simulink subsystem "Colision"  (R2024b)
settings: Solver=VariableStepAuto  StartTime=0.0  StopTime=10.0  RelTol=1e-3
libraries: simulink x4, arduinosensorlib x3
settings Model: Creator=Chenfu  LastModifiedBy=Chenfu

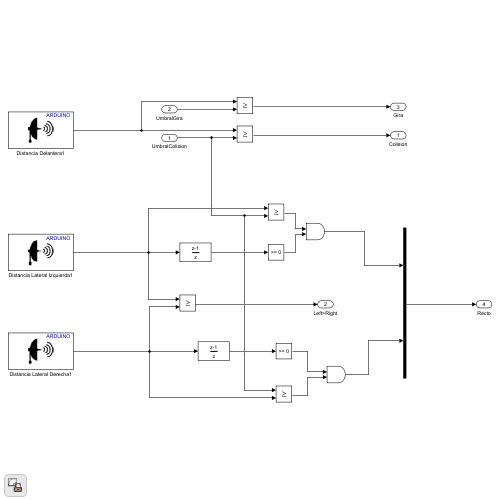
[thumbnail: Simulink's stored preview of the top-level diagram]
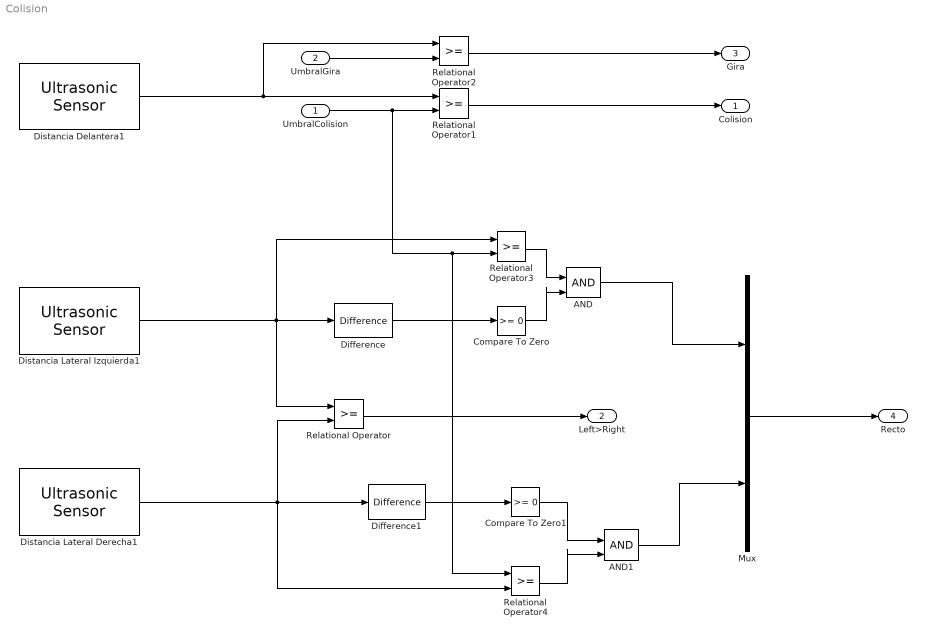
== system Colision ==
  UmbralColision : Inport
  UmbralGira : Inport  Port=2
  AND : Logic  IconShape=distinctive  AllPortsSameDT=off  OutDataTypeStr=boolean
  AND1 : Logic  IconShape=distinctive  AllPortsSameDT=off  OutDataTypeStr=boolean
  Compare To Zero : simulink/Logic and Bit Operations/Compare To Zero  relop=>=  OutDataTypeStr=boolean
  Compare To Zero1 : simulink/Logic and Bit Operations/Compare To Zero  relop=>=  OutDataTypeStr=boolean
  Difference : simulink/Discrete/Difference  ICPrevInput=0.0  OutMin=[]  OutMax=[]  OutDataType=fixdt(1, 16)  OutScaling=2^-10  DoSatur=off
  Difference1 : simulink/Discrete/Difference  ICPrevInput=0.0  OutMin=[]  OutMax=[]  OutDataType=fixdt(1, 16)  OutScaling=2^-10  DoSatur=off
  Distancia Delantera1 : arduinosensorlib/Ultrasonic Sensor  NumSignalPins=2  TrigPin=4  EchoPin=5  SignalPin=3  SampleTime_=0.1  blockPlatform=ARDUINO
  Distancia Lateral Derecha1 : arduinosensorlib/Ultrasonic Sensor  NumSignalPins=2  TrigPin=4  EchoPin=5  SignalPin=3  SampleTime_=0.1  blockPlatform=ARDUINO
  Distancia Lateral Izquierda1 : arduinosensorlib/Ultrasonic Sensor  NumSignalPins=2  TrigPin=4  EchoPin=5  SignalPin=3  SampleTime_=0.1  blockPlatform=ARDUINO
  Mux : Mux  Inputs=2
  Relational Operator{,1..4} (5 alike) : RelationalOperator  OutDataTypeStr=boolean  RndMeth=Simplest  InputSameDT=off
  Colision : Outport
  Left>Right : Outport  Port=2
  Gira : Outport  Port=3
  Recto : Outport  Port=4
  wires:
  Relational Operator/1 -> Left>Right/1
  Distancia Delantera1/1 -> Relational Operator1/1, Relational Operator2/1
  UmbralColision/1 -> Relational Operator1/2, Relational Operator3/2, Relational Operator4/1
  Relational Operator1/1 -> Colision/1
  UmbralGira/1 -> Relational Operator2/2
  Relational Operator2/1 -> Gira/1
  Distancia Lateral Izquierda1/1 -> Relational Operator/1, Difference/1, Relational Operator3/1
  Distancia Lateral Derecha1/1 -> Relational Operator/2, Difference1/1, Relational Operator4/2
  Difference/1 -> Compare To Zero/1
  Compare To Zero/1 -> AND/2
  Relational Operator3/1 -> AND/1
  Difference1/1 -> Compare To Zero1/1
  Relational Operator4/1 -> AND1/2
  Compare To Zero1/1 -> AND1/1
  AND/1 -> Mux/1
  AND1/1 -> Mux/2
  Mux/1 -> Recto/1
